simulink model "MyEngineCU_RTW"  (R2022a)
settings: Solver=ode1  StartTime=0.0  StopTime=inf  FixedStep=0.0002  RelTol=1e-3
PreLoadFcn:
  | vehicle = 'Car'; if ~length(which('cmcmd')), cmenv; end
  | MyEngineCU_RTW_bus
InitFcn:
  | vehicle = 'Car'; if ~length(which('cmcmd')), cmenv; end
  | MyEngineCU_RTW_bus
libraries: simulink x7, CarMaker4SL x3
Description:
  | CarMaker Plug-in Model Target
settings Model: Creator=IPG  LastModifiedBy=IPG
settings SolverCC: AlgebraicLoopSolver=TrustRegion
settings DataIOCC: LimitDataPoints=on  SaveFormat=Array  SignalLoggingSaveFormat=ModelDataLogs  ReturnWorkspaceOutputs=off
settings OptimizationCC: ExpressionDepthLimit=2147483647  LifeSpan=inf
settings DebuggingCC: UnderspecifiedInitializationDetection=Classic  MergeDetectMultiDrivingBlocksExec=none  FcnCallInpInsideContextMsg=warning  UnconnectedInputMsg=warning  UnconnectedOutputMsg=warning  UnconnectedLineMsg=warning  StateNameClashWarn=warning  SFUnexpectedBacktrackingDiag=warning  SFNoUnconditionalDefaultTransitionDiag=warning  SFMachineParentedDataDiag=warning  ArithmeticOperatorsInVariantConditions=warning
settings HardwareCC: ProdBitPerPointer=32  ProdBitPerSizeT=32  ProdBitPerPtrDiffT=32  ProdLargestAtomicFloat=None  ProdIntDivRoundTo=Undefined  ProdEndianess=Unspecified  ProdWordSize=32  ProdHWDeviceType=32-bit Generic  TargetHWDeviceType=32-bit Generic  ProdEqTarget=off
settings ModelReferenceCC: PropagateSignalLabelsOutOfModel=off
settings SFSimCC: SimUseLocalCustomCode=off  CustomCodeUndefinedFunction=UseInterfaceOnly
settings RTWCC: Description=CarMaker Plug-in Model Target  SystemTargetFile=CarMaker.tlc  TemplateMakefile=CarMaker_unix-win64.tmf  RTWUseLocalCustomCode=off  DLArmComputeVersion=19.05
settings CodeAppCC: MaxIdLength=63  StateflowObjectComments=on
settings STFCustomTargetCC: CodeInterfacePackaging=Reusable function  CPPClassGenCompliant=on  GRTInterface=off  GenerateAllocFcn=on  SystemTargetFile=CarMaker.tlc
settings GRTTargetCC: TargetLangStandard=C89/C90 (ANSI)  ParMdlRefBuildCompliant=off  CompOptLevelCompliant=off  ConcurrentExecutionCompliant=off  CombineOutputUpdateFcns=off  MatFileLogging=off  CodeInterfacePackaging=Reusable function  GenerateAllocFcn=on  UseToolchainInfoCompliant=off  ExtModeMexFile=noextcomm
settings ConfigComp: CovMetricSettings=dw  CovSaveCumulativeToWorkspaceVar=on  CovSaveSingleToWorkspaceVar=on  CovExternalEMLEnable=off

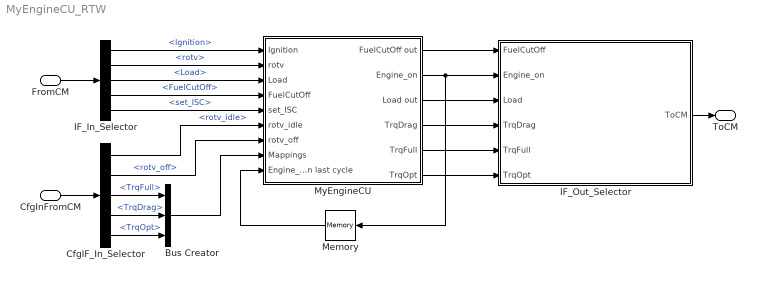
== system MyEngineCU_RTW ==
  FromCM : Inport  OutDataTypeStr=Bus: cmPTEngineCUIn
  CfgInFromCM : Inport  Port=2  OutDataTypeStr=Bus: cmPTEngineCUCfgIn
  Bus Creator : BusCreator  Inputs=3
  CfgIF_In_Selector : BusSelector  OutputSignals=rotv_idle,rotv_off,TrqFull,TrqDrag,TrqOpt
  IF_In_Selector : BusSelector  OutputSignals=Ignition,rotv,Load,FuelCutOff,set_ISC
  IF_Out_Selector : Subsystem  mask(Signal Selection){}
      mask help: Signal Selection Block
      settings: OpenFcn=cmSignalSelect('SignalSelection_CB',gcb)
  Memory : Memory
  MyEngineCU : Subsystem
  ToCM : Outport  OutDataTypeStr=Bus: cmPTEngineCUOut  VectorParamsAs1DForOutWhenUnconnected=off
  wires:
  FromCM/1 -> IF_In_Selector/1
  IF_Out_Selector/1(ToCM) -> ToCM/1
  CfgInFromCM/1 -> CfgIF_In_Selector/1
  IF_In_Selector/1 -> MyEngineCU/1(Ignition)  "<Ignition>"
  IF_In_Selector/2 -> MyEngineCU/2(rotv)  "<rotv>"
  Bus Creator/1 -> MyEngineCU/8(Mappings)
  IF_In_Selector/3 -> MyEngineCU/3(Load)  "<Load>"
  IF_In_Selector/4 -> MyEngineCU/4(FuelCutOff)  "<FuelCutOff>"
  MyEngineCU/1(FuelCutOff out) -> IF_Out_Selector/1(FuelCutOff)
  MyEngineCU/2(Engine_on) -> Memory/1, IF_Out_Selector/2(Engine_on)
  MyEngineCU/3(Load out) -> IF_Out_Selector/3(Load)
  MyEngineCU/4(TrqDrag) -> IF_Out_Selector/4(TrqDrag)
  MyEngineCU/5(TrqFull) -> IF_Out_Selector/5(TrqFull)
  MyEngineCU/6(TrqOpt) -> IF_Out_Selector/6(TrqOpt)
  Memory/1 -> MyEngineCU/9(Engine_on last cycle)
  IF_In_Selector/5 -> MyEngineCU/5(set_ISC)  "<set_ISC>"
  CfgIF_In_Selector/1 -> MyEngineCU/6(rotv_idle)  "<rotv_idle>"
  CfgIF_In_Selector/2 -> MyEngineCU/7(rotv_off)  "<rotv_off>"
  CfgIF_In_Selector/3 -> Bus Creator/1  "<TrqFull>"
  CfgIF_In_Selector/4 -> Bus Creator/2  "<TrqDrag>"
  CfgIF_In_Selector/5 -> Bus Creator/3  "<TrqOpt>"

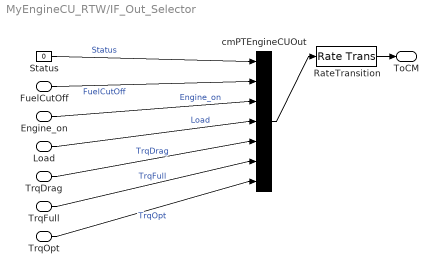
== system MyEngineCU_RTW/IF_Out_Selector ==
  FuelCutOff : Inport
  Engine_on : Inport  Port=2
  Load : Inport  Port=3
  TrqDrag : Inport  Port=4
  TrqFull : Inport  Port=5
  TrqOpt : Inport  Port=6
  RateTransition : RateTransition  OutPortSampleTime=str2num(get_param(bdroot,'FixedStep'))
  Status : Constant  Value=0
  cmPTEngineCUOut : BusCreator  Inputs=7
  ToCM : Outport  VectorParamsAs1DForOutWhenUnconnected=off
  wires:
  RateTransition/1 -> ToCM/1
  cmPTEngineCUOut/1 -> RateTransition/1
  Status/1 -> cmPTEngineCUOut/1  "Status"
  FuelCutOff/1 -> cmPTEngineCUOut/2  "FuelCutOff"
  Engine_on/1 -> cmPTEngineCUOut/3  "Engine_on"
  Load/1 -> cmPTEngineCUOut/4  "Load"
  TrqDrag/1 -> cmPTEngineCUOut/5  "TrqDrag"
  TrqFull/1 -> cmPTEngineCUOut/6  "TrqFull"
  TrqOpt/1 -> cmPTEngineCUOut/7  "TrqOpt"

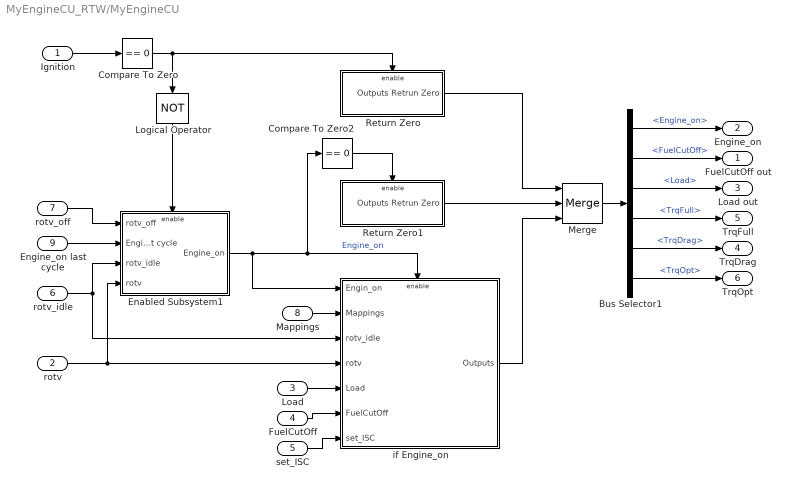
== system MyEngineCU_RTW/MyEngineCU ==
  Ignition : Inport
  rotv : Inport  Port=2
  Load : Inport  Port=3
  FuelCutOff : Inport  Port=4
  set_ISC : Inport  Port=5
  rotv_idle : Inport  Port=6
  rotv_off : Inport  Port=7
  Mappings : Inport  Port=8
  Engine_on last cycle : Inport  Port=9
  Bus Selector1 : BusSelector  OutputSignals=Engine_on,FuelCutOff,Load,TrqFull,TrqDrag,TrqOpt
  Compare To Zero : simulink/Logic and Bit Operations/Compare To Zero  relop===  OutDataTypeStr=uint8  ZeroCross=off
  Compare To Zero2 : simulink/Logic and Bit Operations/Compare To Zero  relop===  OutDataTypeStr=uint8  ZeroCross=off
  Enabled Subsystem1 : Subsystem  TreatAsAtomicUnit=on
  Logical Operator : Logic  Operator=NOT  AllPortsSameDT=off  OutDataTypeStr=boolean
  Merge : Merge  Inputs=3
  Return Zero : Subsystem  TreatAsAtomicUnit=on
  Return Zero1 : Subsystem  TreatAsAtomicUnit=on
  if Engine_on : Subsystem  TreatAsAtomicUnit=on
  FuelCutOff out : Outport  VectorParamsAs1DForOutWhenUnconnected=off
  Engine_on : Outport  Port=2  VectorParamsAs1DForOutWhenUnconnected=off
  Load out : Outport  Port=3  VectorParamsAs1DForOutWhenUnconnected=off
  TrqDrag : Outport  Port=4  VectorParamsAs1DForOutWhenUnconnected=off
  TrqFull : Outport  Port=5  VectorParamsAs1DForOutWhenUnconnected=off
  TrqOpt : Outport  Port=6  VectorParamsAs1DForOutWhenUnconnected=off
  wires:
  Ignition/1 -> Compare To Zero/1
  Compare To Zero/1 -> Logical Operator/1, Return Zero/Enable
  Logical Operator/1 -> Enabled Subsystem1/Enable
  Enabled Subsystem1/1(Engine_on) -> Compare To Zero2/1, if Engine_on/Enable, if Engine_on/1(Engin_on)  "Engine_on"
  Mappings/1 -> if Engine_on/2(Mappings)
  rotv/1 -> Enabled Subsystem1/4(rotv), if Engine_on/4(rotv)
  rotv_idle/1 -> Enabled Subsystem1/3(rotv_idle), if Engine_on/3(rotv_idle)
  rotv_off/1 -> Enabled Subsystem1/1(rotv_off)
  Engine_on last cycle/1 -> Enabled Subsystem1/2(Engine_on last cycle)
  Load/1 -> if Engine_on/5(Load)
  FuelCutOff/1 -> if Engine_on/6(FuelCutOff)
  set_ISC/1 -> if Engine_on/7(set_ISC)
  Return Zero/1(Outputs Retrun Zero) -> Merge/1
  Merge/1 -> Bus Selector1/1
  Bus Selector1/1 -> Engine_on/1  "<Engine_on>"
  Bus Selector1/3 -> Load out/1  "<Load>"
  Bus Selector1/5 -> TrqDrag/1  "<TrqDrag>"
  Bus Selector1/4 -> TrqFull/1  "<TrqFull>"
  Bus Selector1/6 -> TrqOpt/1  "<TrqOpt>"
  Bus Selector1/2 -> FuelCutOff out/1  "<FuelCutOff>"
  Compare To Zero2/1 -> Return Zero1/Enable
  Return Zero1/1(Outputs Retrun Zero) -> Merge/2
  if Engine_on/1(Outputs) -> Merge/3

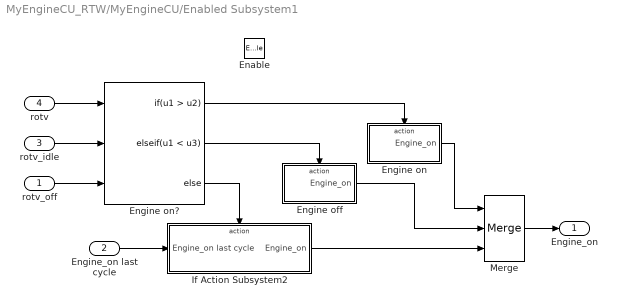
== system MyEngineCU_RTW/MyEngineCU/Enabled Subsystem1 ==
  rotv_off : Inport
  Engine_on last cycle : Inport  Port=2
  rotv_idle : Inport  Port=3
  rotv : Inport  Port=4
  Enable : EnablePort
  Engine off : Subsystem  TreatAsAtomicUnit=on
  Engine on : Subsystem  TreatAsAtomicUnit=on
  Engine on? : If  NumInputs=3  IfExpression=u1 > u2  ElseIfExpressions=u1 < u3
  If Action Subsystem2 : Subsystem  TreatAsAtomicUnit=on
  Merge : Merge  Inputs=3
  Engine_on : Outport  VectorParamsAs1DForOutWhenUnconnected=off
  wires:
  rotv/1 -> Engine on?/1
  rotv_idle/1 -> Engine on?/2
  rotv_off/1 -> Engine on?/3
  Engine on?/1 -> Engine on/Action
  Engine on?/2 -> Engine off/Action
  Engine on?/3 -> If Action Subsystem2/Action
  Engine_on last cycle/1 -> If Action Subsystem2/1(Engine_on last cycle)
  Merge/1 -> Engine_on/1
  If Action Subsystem2/1(Engine_on) -> Merge/3
  Engine on/1(Engine_on) -> Merge/1
  Engine off/1(Engine_on) -> Merge/2

== system MyEngineCU_RTW/MyEngineCU/Return Zero ==
  Enable : EnablePort
  Bus Creator : BusCreator  Inputs=6
  Constant : Constant  Value=0
  Constant1 : Constant  Value=0
  Constant{2..5} (4 alike) : Constant  Value=0.0
  Outputs Retrun Zero : Outport  InitialOutput=0  VectorParamsAs1DForOutWhenUnconnected=off
  wires:
  Bus Creator/1 -> Outputs Retrun Zero/1
  Constant/1 -> Bus Creator/1  "Engine_on"
  Constant1/1 -> Bus Creator/2  "FuelCutOff"
  Constant2/1 -> Bus Creator/3  "Load"
  Constant3/1 -> Bus Creator/4  "TrqFull"
  Constant4/1 -> Bus Creator/5  "TrqDrag"
  Constant5/1 -> Bus Creator/6  "TrqOpt"

== system MyEngineCU_RTW/MyEngineCU/Return Zero1 ==
  Enable : EnablePort
  Bus Creator : BusCreator  Inputs=6
  Constant : Constant  Value=0
  Constant1 : Constant  Value=0
  Constant{2..5} (4 alike) : Constant  Value=0.0
  Outputs Retrun Zero : Outport  InitialOutput=0  VectorParamsAs1DForOutWhenUnconnected=off
  wires:
  Constant5/1 -> Bus Creator/6  "TrqOpt"
  Constant4/1 -> Bus Creator/5  "TrqDrag"
  Constant3/1 -> Bus Creator/4  "TrqFull"
  Constant2/1 -> Bus Creator/3  "Load"
  Constant1/1 -> Bus Creator/2  "FuelCutOff"
  Constant/1 -> Bus Creator/1  "Engine_on"
  Bus Creator/1 -> Outputs Retrun Zero/1

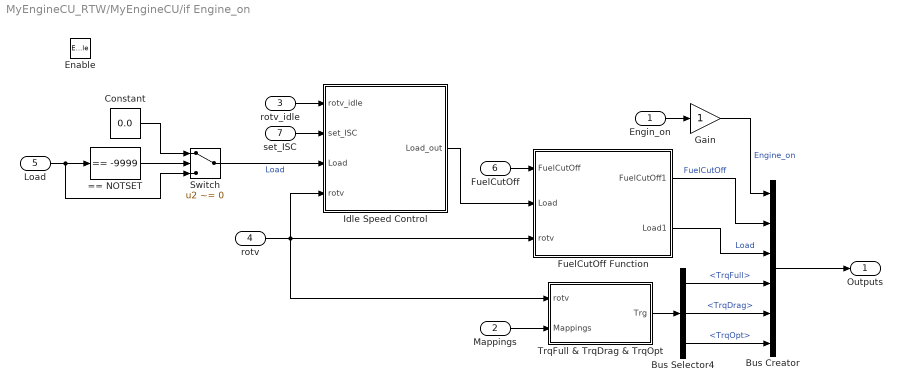
== system MyEngineCU_RTW/MyEngineCU/if Engine_on ==
  Engin_on : Inport
  Mappings : Inport  Port=2
  rotv_idle : Inport  Port=3
  rotv : Inport  Port=4
  Load : Inport  Port=5
  FuelCutOff : Inport  Port=6
  set_ISC : Inport  Port=7
  Enable : EnablePort
  == NOTSET : simulink/Logic and Bit Operations/Compare To Constant  relop===  const=-9999  OutDataTypeStr=uint8  ZeroCross=off
  Bus Creator : BusCreator  Inputs=6
  Bus Selector4 : BusSelector  OutputSignals=TrqFull,TrqDrag,TrqOpt
  Constant : Constant  Value=0.0
  FuelCutOff Function : Subsystem
  Gain : Gain
  Idle Speed Control : Subsystem
  Switch : Switch  Criteria=u2 ~= 0  SaturateOnIntegerOverflow=off  InputSameDT=off
  TrqFull & TrqDrag & TrqOpt : Subsystem
  Outputs : Outport  VectorParamsAs1DForOutWhenUnconnected=off
  wires:
  Bus Creator/1 -> Outputs/1
  Mappings/1 -> TrqFull & TrqDrag & TrqOpt/2(Mappings)
  rotv/1 -> FuelCutOff Function/3(rotv), Idle Speed Control/4(rotv), TrqFull & TrqDrag & TrqOpt/1(rotv)
  Load/1 -> == NOTSET/1, Switch/3
  == NOTSET/1 -> Switch/2
  Constant/1 -> Switch/1
  TrqFull & TrqDrag & TrqOpt/1(Trg) -> Bus Selector4/1
  FuelCutOff/1 -> FuelCutOff Function/1(FuelCutOff)
  Idle Speed Control/1(Load_out) -> FuelCutOff Function/2(Load)
  rotv_idle/1 -> Idle Speed Control/1(rotv_idle)
  set_ISC/1 -> Idle Speed Control/2(set_ISC)
  Switch/1 -> Idle Speed Control/3(Load)  "Load"
  Engin_on/1 -> Gain/1
  FuelCutOff Function/1(FuelCutOff1) -> Bus Creator/2  "FuelCutOff"
  FuelCutOff Function/2(Load1) -> Bus Creator/3  "Load"
  Bus Selector4/1 -> Bus Creator/4  "<TrqFull>"
  Bus Selector4/2 -> Bus Creator/5  "<TrqDrag>"
  Bus Selector4/3 -> Bus Creator/6  "<TrqOpt>"
  Gain/1 -> Bus Creator/1  "Engine_on"

== system MyEngineCU_RTW/MyEngineCU/Enabled Subsystem1/Engine off ==
  Action Port : ActionPort  ActionPortLabel=elseif { }
  Constant : Constant  Value=0
  Engine_on : Outport  InitialOutput=0  VectorParamsAs1DForOutWhenUnconnected=off
  wires:
  Constant/1 -> Engine_on/1

== system MyEngineCU_RTW/MyEngineCU/Enabled Subsystem1/Engine on ==
  Action Port : ActionPort  ActionPortLabel=if { }
  Constant : Constant
  Engine_on : Outport  InitialOutput=1  VectorParamsAs1DForOutWhenUnconnected=off
  wires:
  Constant/1 -> Engine_on/1

== system MyEngineCU_RTW/MyEngineCU/Enabled Subsystem1/If Action Subsystem2 ==
  Engine_on last cycle : Inport
  Action Port : ActionPort  ActionPortLabel=else { }
  Engine_on : Outport  VectorParamsAs1DForOutWhenUnconnected=off
  wires:
  Engine_on last cycle/1 -> Engine_on/1

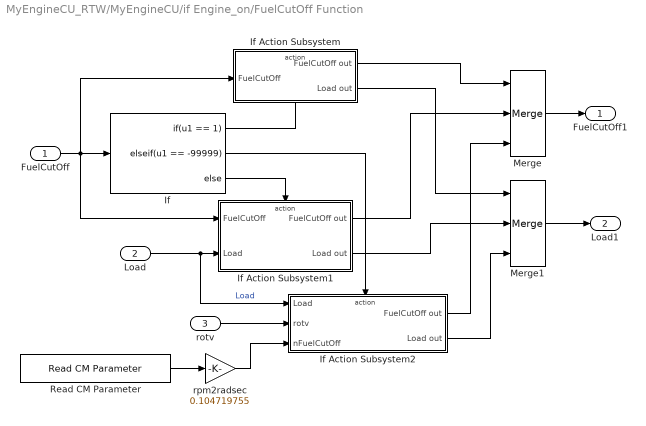
== system MyEngineCU_RTW/MyEngineCU/if Engine_on/FuelCutOff Function ==
  FuelCutOff : Inport
  Load : Inport  Port=2
  rotv : Inport  Port=3
  If : If  IfExpression=u1 == 1  ElseIfExpressions=u1 == -99999
  If Action Subsystem : Subsystem  TreatAsAtomicUnit=on
  If Action Subsystem1 : Subsystem  TreatAsAtomicUnit=on
  If Action Subsystem2 : Subsystem  TreatAsAtomicUnit=on
  Merge : Merge  Inputs=3
  Merge1 : Merge  Inputs=3
  Read CM Parameter : CarMaker4SL/Read CM Parameter  xfile=Vehicle  xkey=PowerTrain.ECU.FuelCutOff  xnout=1  xdefaults=1600  xmuxed=on
      settings: SourceProductName=CarMaker4SL
  rpm2radsec : Gain  Gain=0.104719755
  FuelCutOff1 : Outport  VectorParamsAs1DForOutWhenUnconnected=off
  Load1 : Outport  Port=2  VectorParamsAs1DForOutWhenUnconnected=off
  wires:
  If/3 -> If Action Subsystem1/Action
  If/2 -> If Action Subsystem2/Action
  If/1 -> If Action Subsystem/Action
  If Action Subsystem/1(FuelCutOff out) -> Merge/1
  If Action Subsystem1/1(FuelCutOff out) -> Merge/2
  If Action Subsystem2/1(FuelCutOff out) -> Merge/3
  If Action Subsystem2/2(Load out) -> Merge1/3
  If Action Subsystem1/2(Load out) -> Merge1/2
  If Action Subsystem/2(Load out) -> Merge1/1
  rotv/1 -> If Action Subsystem2/2(rotv)
  Read CM Parameter/1 -> rpm2radsec/1
  Merge/1 -> FuelCutOff1/1
  Merge1/1 -> Load1/1
  FuelCutOff/1 -> If/1, If Action Subsystem/1(FuelCutOff), If Action Subsystem1/1(FuelCutOff)
  Load/1 -> If Action Subsystem1/2(Load), If Action Subsystem2/1(Load)  "Load"
  rpm2radsec/1 -> If Action Subsystem2/3(nFuelCutOff)

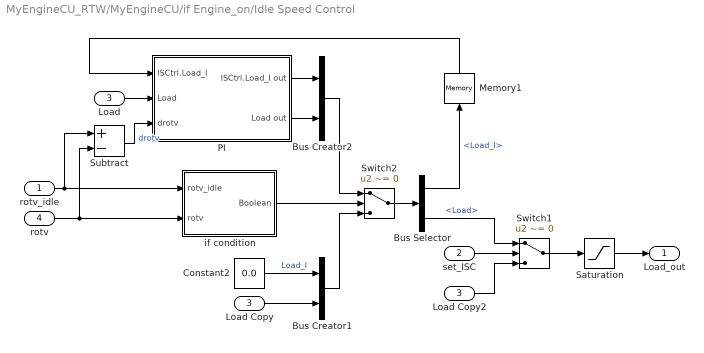
== system MyEngineCU_RTW/MyEngineCU/if Engine_on/Idle Speed Control ==
  rotv_idle : Inport
  set_ISC : Inport  Port=2
  Load : Inport  Port=3
  rotv : Inport  Port=4
  Bus Creator1 : BusCreator  Inputs=2
  Bus Creator2 : BusCreator  Inputs=2
  Bus Selector : BusSelector  OutputSignals=Load_I,Load
  Constant2 : Constant  Value=0.0
  Load Copy : InportShadow  Port=3
  Load Copy2 : InportShadow  Port=3
  Memory1 : Memory  InheritSampleTime=on
  PI : Subsystem
  Saturation : Saturate  UpperLimit=1  LowerLimit=0
  Subtract : Sum  Inputs=+-
  Switch1 : Switch  Criteria=u2 ~= 0  SaturateOnIntegerOverflow=off  InputSameDT=off
  Switch2 : Switch  Criteria=u2 ~= 0  SaturateOnIntegerOverflow=off  InputSameDT=off
  if condition : Subsystem
  Load_out : Outport  VectorParamsAs1DForOutWhenUnconnected=off
  wires:
  Switch1/1 -> Saturation/1
  Load/1 -> PI/2(Load)
  set_ISC/1 -> Switch1/2
  Switch2/1 -> Bus Selector/1
  Bus Creator1/1 -> Switch2/3
  Bus Creator2/1 -> Switch2/1
  if condition/1(Boolean) -> Switch2/2
  Constant2/1 -> Bus Creator1/1  "Load_I"
  Saturation/1 -> Load_out/1
  rotv_idle/1 -> if condition/1(rotv_idle), Subtract/1
  rotv/1 -> if condition/2(rotv), Subtract/2
  PI/1(ISCtrl.Load_I out) -> Bus Creator2/1
  Bus Selector/2 -> Switch1/1  "<Load>"
  Bus Selector/1 -> Memory1/1  "<Load_I>"
  Memory1/1 -> PI/1(ISCtrl.Load_I)
  Subtract/1 -> PI/3(drotv)  "drotv"
  PI/2(Load out) -> Bus Creator2/2
  Load Copy/1 -> Bus Creator1/2
  Load Copy2/1 -> Switch1/3

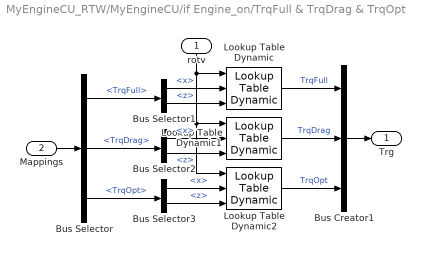
== system MyEngineCU_RTW/MyEngineCU/if Engine_on/TrqFull & TrqDrag & TrqOpt ==
  rotv : Inport
  Mappings : Inport  Port=2
  Bus Creator1 : BusCreator  Inputs=3
  Bus Selector : BusSelector  OutputSignals=TrqFull,TrqDrag,TrqOpt
  Bus Selector1 : BusSelector  OutputSignals=x,z
  Bus Selector2 : BusSelector  OutputSignals=x,z
  Bus Selector3 : BusSelector  OutputSignals=x,z
  Lookup Table Dynamic : simulink/Lookup Tables/Lookup Table Dynamic  LookUpMeth=Interpolation-Use End Values  OutDataTypeStr=float('double')  OutputDataTypeScalingMode=Specify via dialog  OutDataType=float('double')  OutScaling=2^-10  DoSatur=off
  Lookup Table Dynamic1 : simulink/Lookup Tables/Lookup Table Dynamic  LookUpMeth=Interpolation-Use End Values  OutDataTypeStr=float('double')  OutputDataTypeScalingMode=Specify via dialog  OutDataType=float('double')  OutScaling=2^-10  DoSatur=off
  Lookup Table Dynamic2 : simulink/Lookup Tables/Lookup Table Dynamic  LookUpMeth=Interpolation-Use End Values  OutDataTypeStr=float('double')  OutputDataTypeScalingMode=Specify via dialog  OutDataType=float('double')  OutScaling=2^-10  DoSatur=off
  Trg : Outport  VectorParamsAs1DForOutWhenUnconnected=off
  wires:
  Bus Selector1/1 -> Lookup Table Dynamic/2  "<x>"
  Bus Selector1/2 -> Lookup Table Dynamic/3  "<z>"
  Bus Selector/1 -> Bus Selector1/1  "<TrqFull>"
  Bus Selector/2 -> Bus Selector2/1  "<TrqDrag>"
  Bus Selector/3 -> Bus Selector3/1  "<TrqOpt>"
  Bus Selector2/2 -> Lookup Table Dynamic1/3  "<z>"
  Bus Selector2/1 -> Lookup Table Dynamic1/2  "<x>"
  Bus Selector3/1 -> Lookup Table Dynamic2/2  "<x>"
  Bus Selector3/2 -> Lookup Table Dynamic2/3  "<z>"
  Lookup Table Dynamic/1 -> Bus Creator1/1  "TrqFull"
  Lookup Table Dynamic1/1 -> Bus Creator1/2  "TrqDrag"
  Lookup Table Dynamic2/1 -> Bus Creator1/3  "TrqOpt"
  rotv/1 -> Lookup Table Dynamic/1, Lookup Table Dynamic1/1, Lookup Table Dynamic2/1
  Bus Creator1/1 -> Trg/1
  Mappings/1 -> Bus Selector/1

== system MyEngineCU_RTW/MyEngineCU/if Engine_on/FuelCutOff Function/If Action Subsystem ==
  FuelCutOff : Inport
  Action Port : ActionPort  ActionPortLabel=if { }
  Constant : Constant  Value=0.0
  FuelCutOff out : Outport  VectorParamsAs1DForOutWhenUnconnected=off
  Load out : Outport  Port=2  InitialOutput=0  VectorParamsAs1DForOutWhenUnconnected=off
  wires:
  Constant/1 -> Load out/1
  FuelCutOff/1 -> FuelCutOff out/1

== system MyEngineCU_RTW/MyEngineCU/if Engine_on/FuelCutOff Function/If Action Subsystem1 ==
  FuelCutOff : Inport
  Load : Inport  Port=2
  Action Port : ActionPort  ActionPortLabel=else { }
  FuelCutOff out : Outport  VectorParamsAs1DForOutWhenUnconnected=off
  Load out : Outport  Port=2  VectorParamsAs1DForOutWhenUnconnected=off
  wires:
  Load/1 -> Load out/1
  FuelCutOff/1 -> FuelCutOff out/1

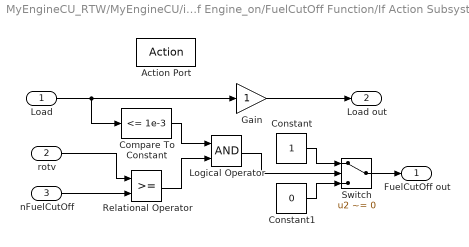
== system MyEngineCU_RTW/MyEngineCU/if Engine_on/FuelCutOff Function/If Action Subsystem2 ==
  Load : Inport
  rotv : Inport  Port=2
  nFuelCutOff : Inport  Port=3
  Action Port : ActionPort  ActionPortLabel=elseif { }
  Compare To Constant : simulink/Logic and Bit Operations/Compare To Constant  relop=<=  const=1e-3  OutDataTypeStr=uint8  ZeroCross=off
  Constant : Constant
  Constant1 : Constant  Value=0
  Gain : Gain
  Logical Operator : Logic  AllPortsSameDT=off  OutDataTypeStr=boolean
  Relational Operator : RelationalOperator  OutDataTypeStr=boolean  InputSameDT=off
  Switch : Switch  Criteria=u2 ~= 0  SaturateOnIntegerOverflow=off  InputSameDT=off
  FuelCutOff out : Outport  VectorParamsAs1DForOutWhenUnconnected=off
  Load out : Outport  Port=2  VectorParamsAs1DForOutWhenUnconnected=off
  wires:
  Load/1 -> Compare To Constant/1, Gain/1
  Switch/1 -> FuelCutOff out/1
  rotv/1 -> Relational Operator/1
  nFuelCutOff/1 -> Relational Operator/2
  Relational Operator/1 -> Logical Operator/2
  Compare To Constant/1 -> Logical Operator/1
  Logical Operator/1 -> Switch/2
  Constant/1 -> Switch/1
  Constant1/1 -> Switch/3
  Gain/1 -> Load out/1

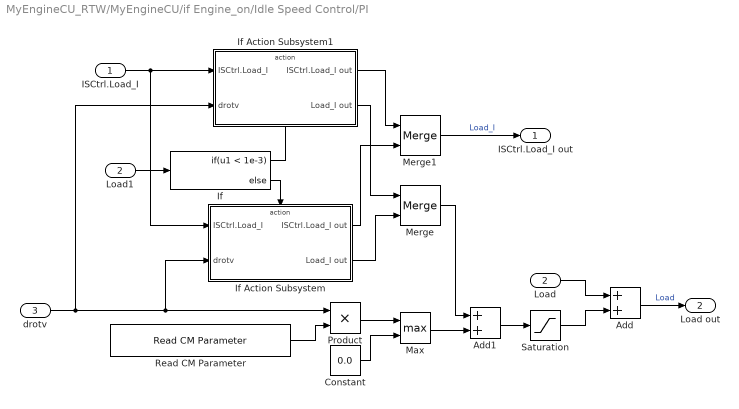
== system MyEngineCU_RTW/MyEngineCU/if Engine_on/Idle Speed Control/PI ==
  ISCtrl.Load_I : Inport
  Load : Inport  Port=2
  drotv : Inport  Port=3
  Add : Sum
  Add1 : Sum
  Constant : Constant  Value=0.0
  If : If  IfExpression=u1 < 1e-3
  If Action Subsystem : Subsystem  TreatAsAtomicUnit=on
  If Action Subsystem1 : Subsystem  TreatAsAtomicUnit=on
  Load1 : InportShadow  Port=2
  Max : MinMax  Function=max  Inputs=2
  Merge : Merge
  Merge1 : Merge
  Product : Product  RndMeth=Zero
  Read CM Parameter : CarMaker4SL/Read CM Parameter  xfile=Vehicle  xkey=PowerTrain.MyEngineCU.ISCtrl.P  xnout=1  xdefaults=0.1  xmuxed=on
      settings: SourceProductName=CarMaker4SL
  Saturation : Saturate  UpperLimit=1  LowerLimit=0
  ISCtrl.Load_I out : Outport  VectorParamsAs1DForOutWhenUnconnected=off
  Load out : Outport  Port=2  VectorParamsAs1DForOutWhenUnconnected=off
  wires:
  Add/1 -> Load out/1  "Load"
  Add1/1 -> Saturation/1
  drotv/1 -> Product/1, If Action Subsystem/2(drotv), If Action Subsystem1/2(drotv)
  Read CM Parameter/1 -> Product/2
  Product/1 -> Max/1
  Max/1 -> Add1/2
  Constant/1 -> Max/2
  Load/1 -> Add/1
  ISCtrl.Load_I/1 -> If Action Subsystem/1(ISCtrl.Load_I), If Action Subsystem1/1(ISCtrl.Load_I)
  If/2 -> If Action Subsystem/Action
  Merge/1 -> Add1/1
  If Action Subsystem/2(Load_I out) -> Merge/2
  If Action Subsystem/1(ISCtrl.Load_I out) -> Merge1/2
  If/1 -> If Action Subsystem1/Action
  If Action Subsystem1/2(Load_I out) -> Merge/1
  If Action Subsystem1/1(ISCtrl.Load_I out) -> Merge1/1
  Merge1/1 -> ISCtrl.Load_I out/1  "Load_I"
  Load1/1 -> If/1
  Saturation/1 -> Add/2

== system MyEngineCU_RTW/MyEngineCU/if Engine_on/Idle Speed Control/if condition ==
  rotv_idle : Inport
  rotv : Inport  Port=2
  Add : Sum
  Constant1 : Constant  Value=200.0
  Relational Operator : RelationalOperator  Operator=<  OutDataTypeStr=boolean  InputSameDT=off
  rpm2radsec : Gain  Gain=0.104719755
  Boolean : Outport  VectorParamsAs1DForOutWhenUnconnected=off
  wires:
  rpm2radsec/1 -> Add/2
  Constant1/1 -> rpm2radsec/1
  rotv_idle/1 -> Add/1
  Relational Operator/1 -> Boolean/1
  rotv/1 -> Relational Operator/1
  Add/1 -> Relational Operator/2

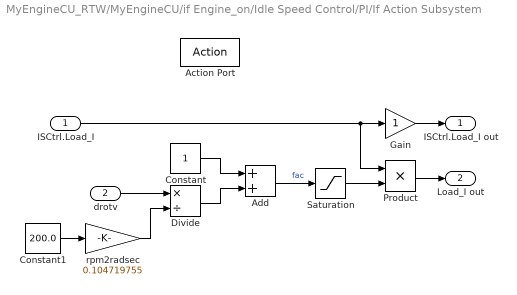
== system MyEngineCU_RTW/MyEngineCU/if Engine_on/Idle Speed Control/PI/If Action Subsystem ==
  ISCtrl.Load_I : Inport
  drotv : Inport  Port=2
  Action Port : ActionPort  ActionPortLabel=else { }
  Add : Sum
  Constant : Constant
  Constant1 : Constant  Value=200.0
  Divide : Product  Inputs=*/
  Gain : Gain
  Product : Product  RndMeth=Zero
  Saturation : Saturate  UpperLimit=1  LowerLimit=0
  rpm2radsec : Gain  Gain=0.104719755
  ISCtrl.Load_I out : Outport  VectorParamsAs1DForOutWhenUnconnected=off
  Load_I out : Outport  Port=2  VectorParamsAs1DForOutWhenUnconnected=off
  wires:
  ISCtrl.Load_I/1 -> Product/1, Gain/1
  Product/1 -> Load_I out/1
  Add/1 -> Saturation/1  "fac"
  Constant/1 -> Add/1
  Divide/1 -> Add/2
  drotv/1 -> Divide/1
  rpm2radsec/1 -> Divide/2
  Constant1/1 -> rpm2radsec/1
  Saturation/1 -> Product/2
  Gain/1 -> ISCtrl.Load_I out/1

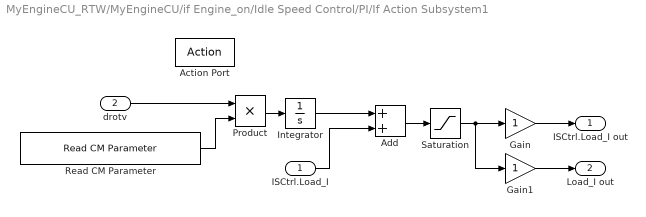
== system MyEngineCU_RTW/MyEngineCU/if Engine_on/Idle Speed Control/PI/If Action Subsystem1 ==
  ISCtrl.Load_I : Inport
  drotv : Inport  Port=2
  Action Port : ActionPort  ActionPortLabel=if { }
  Add : Sum
  Gain : Gain
  Gain1 : Gain
  Integrator : Integrator
  Product : Product  RndMeth=Zero
  Read CM Parameter : CarMaker4SL/Read CM Parameter  xfile=Vehicle  xkey=PowerTrain.MyEngineCU.ISCtrl.I  xnout=1  xdefaults=[]  xmuxed=on
      settings: SourceProductName=CarMaker4SL
  Saturation : Saturate  UpperLimit=1  LowerLimit=0
  ISCtrl.Load_I out : Outport  VectorParamsAs1DForOutWhenUnconnected=off
  Load_I out : Outport  Port=2  VectorParamsAs1DForOutWhenUnconnected=off
  wires:
  Add/1 -> Saturation/1
  Saturation/1 -> Gain/1, Gain1/1
  ISCtrl.Load_I/1 -> Add/2
  Product/1 -> Integrator/1
  drotv/1 -> Product/1
  Read CM Parameter/1 -> Product/2
  Gain/1 -> ISCtrl.Load_I out/1
  Gain1/1 -> Load_I out/1
  Integrator/1 -> Add/1
